simulink model "CR"  (R2022a)
settings: Solver=FixedStepDiscrete  StartTime=0.0  StopTime=1  FixedStep=0.04  RelTol=1e-3
PreLoadFcn:
  | listing = dir;
  | if (contains([listing .name], 'AGR')) && (contains([listing .name], 'MAP'))
  |     addpath('./AGR', './MAP');
  |     addpath( genpath('./MAP') );
  | elseif (contains([listing .name], 'CR.slx'))
  |     addpath('../AGR', '../MAP');
  |     addpath( genpath('../MAP') );
  | else
  | 
  | end
  | 
  | load('BusStructureCR.mat');
InitFcn:
  | listing = dir;
  | if (contains([listing .name], 'AGR')) && (contains([listing .name], 'MAP'))
  |     addpath('./AGR', './MAP');
  |     addpath( genpath('./MAP') );
  | elseif (contains([listing .name], 'CR.slx'))
  |     addpath('../AGR', '../MAP');
  |     addpath( genpath('../MAP') );
  | else
  | 
  | end
  | 
  | load('BusStructureCR.mat');
StartFcn:
  | listing = dir;
  | if (contains([listing .name], 'AGR')) && (contains([listing .name], 'MAP'))
  |     addpath('./AGR', './MAP');
  |     addpath( genpath('./MAP') );
  | elseif (contains([listing .name], 'CR.slx'))
  |     addpath('../AGR', '../MAP');
  |     addpath( genpath('../MAP') );
  | else
  | 
  | end
  | 
  | load('BusStructureCR.mat');
undefined symbols (not defined in the file or in its folder): CRDataTag, CRDataTagWrap, CRElevationValid, CRSelected, CRSelectedWraparound, CRTargetElevation, CRTargetLatitude, CRTargetLongitude, CRTargetLOSAvailable, CRTargetLOSAvailableValid, CRValid, deltaECEF, isFeasible, llh, losECEF, nSearch, targetECEF, testLLH
libraries: aerolibconvert2 x1
settings Model: Creator=ASCL  LastModifiedBy=ASCL
settings DataIOCC: SaveOutput=off  SignalLogging=off  DSMLogging=off  SaveTime=off  ReturnWorkspaceOutputs=off
settings OptimizationCC: BlockReduction=off  DefaultParameterBehavior=Inlined  UseDivisionForNetSlopeComputation=on  GainParamInheritBuiltInType=on  UseFloatMulNetSlope=on  ExpressionFolding=off  PassReuseOutputArgsAs=Individual arguments  ZeroExternalMemoryAtStartup=off  ZeroInternalMemoryAtStartup=off  NoFixptDivByZeroProtection=on  EfficientFloat2IntCast=on  LifeSpan=inf  OptimizeBlockOrder=speed  DifferentSizesBufferReuse=on  EfficientTunableParamExpr=on
settings DebuggingCC: SignalInfNanChecking=warning  ReadBeforeWriteMsg=EnableAllAsWarning  WriteAfterWriteMsg=EnableAllAsError  WriteAfterReadMsg=EnableAllAsError  IntegerOverflowMsg=error  ParameterTunabilityLossMsg=error  UniqueDataStoreMsg=error  AssertControl=DisableAll  NonBusSignalsTreatedAsBus=error  SFInvalidInputDataAccessInChartInitDiag=error  SFTransitionOutsideNaturalParentDiag=error  SFUnreachableExecutionPathDiag=error  SFUndirectedBroadcastEventsDiag=error  IntegerSaturationMsg=error
settings HardwareCC: ProdBitPerPointer=32  ProdBitPerSizeT=32  ProdBitPerPtrDiffT=32  ProdLargestAtomicInteger=Long  ProdLargestAtomicFloat=Double  ProdEndianess=BigEndian  ProdWordSize=32  ProdLongLongMode=on  ProdHWDeviceType=Freescale->MPC83xx
settings ModelReferenceCC: ModelReferenceNumInstancesAllowed=Single
settings SFSimCC: SimCustomHeaderCode="#include \"MAP.h\""  SimUserSources=MAP.c  SimUserLibraries=WS2_32.LIB  CompileTimeRecursionLimit=0  EnableRuntimeRecursion=off  MATLABDynamicMemAlloc=off
settings RTWCC: SystemTargetFile=ert.tlc  TemplateMakefile=ert_default_tmf  GenerateReport=on  RTWUseSimCustomCode=on  CustomHeaderCode="#include \"MAP.h\""  CustomSource=MAP.c  CustomLibrary=WS2_32.LIB  BuildConfiguration=Faster Runs  IncludeHyperlinkInReport=on  LaunchReport=on  GenerateTraceInfo=on  GenerateTraceReport=on  GenerateTraceReportSl=on  GenerateTraceReportSf=on  GenerateTraceReportEml=on  GenerateCodeMetricsReport=on
settings CodeAppCC: ForceParamTrailComments=on  IgnoreCustomStorageClasses=off  OperatorAnnotations=on  SimulinkDataObjDesc=on  SFDataObjDesc=on  MATLABFcnDesc=on  InsertBlockDesc=on  StateflowObjectComments=on  MATLABSourceComments=on  EnableCustomComments=on  InlinedPrmAccess=Macros  ReqsInCode=on
settings ERTTargetCC: TargetLangStandard=C99 (ISO)  UtilityFuncGeneration=Shared location  GenerateSampleERTMain=on  IncludeMdlTerminateFcn=off  CombineSignalStateStructs=on  SuppressErrorStatus=on  SupportAbsoluteTime=off  SupportNonFinite=off  SupportComplex=off  SupportVariableSizeSignals=on  ParenthesesLevel=Standards  CastingMode=Standards  GenerateSharedConstants=off  InlinedParameterPlacement=NonHierarchical  ERTCustomFileTemplate=example_file_process.tlc  RateTransitionBlockCode=Function  PreserveIfCondition=on  ConvertIfToSwitch=off  EnableSignedLeftShifts=off  EnableSignedRightShifts=off

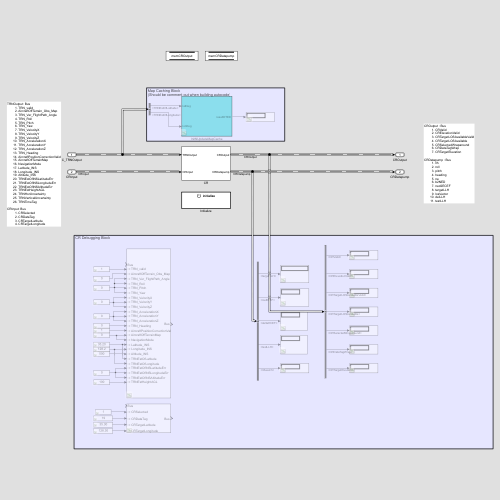
[thumbnail: Simulink's stored preview of the top-level diagram]
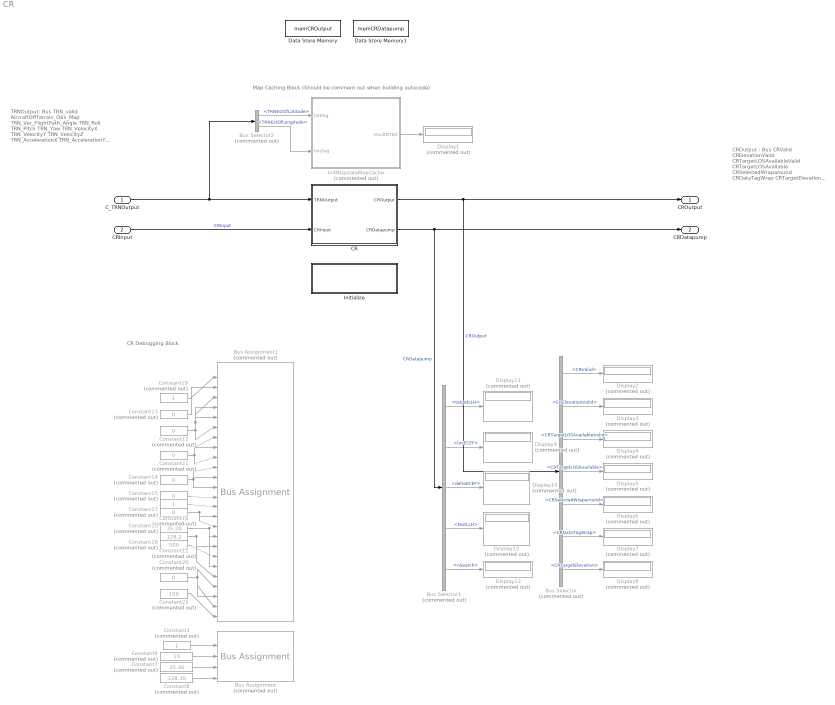
== system CR ==
  note: Map Caching Block
      | (Should be comment out when building autocode)
  note: TRNOutput: Bus
      | TRN_valid
      | AircraftOffTerrain_Obs_Map
      | TRN_Ver_FlightPath_Angle
      | TRN_Roll
      | TRN_Pitch
      | TRN_Yaw
      | TRN_VelocityX
      | TRN_VelocityY
      | TRN_VelocityZ
      | TRN_AccelerationX
      | TRN_AccelerationY
      | TRN_AccelerationZ
      | TRN_Heading
      | AircraftPositionCorrectionValid
      | AircraftOffTerrainMap
      | NavigationMode
      | Latitude_INS
      | Longitude_INS
      | Altitude_INS
      | TRNEstOfINSLatitudeErr
      | TRNEstOfINSLongitudeErr
      | TRNEstOfINSAltitudeErr
      | TRNEstHeightAGL
      | TRNHorUncertainty
      | TRNVerticalUncertainty
      | TRNTimeTag
      |
      | CRInput: Bus
      | CRSelected
      | CRDataTag
      | CRTargetLatitude
      | CRTargetLongitude
  note: CROutput : Bus
      | CRValid
      | CRElevationValid
      | CRTargetLOSAvailableValid
      | CRTargetLOSAvailable
      | CRSelectedWraparound
      | CRDataTagWrap
      | CRTargetElevation
      |
      | CRDatapump : Bus
      | llh
      | roll
      | pitch
      | heading
      | ne
      | b2NED
      | ned2ECEF
      | targetLLH
      | losVector
      | delLLH
      | testLLH
  note: CR Debugging Block
  C_TRNOutput : Inport  OutDataTypeStr=Bus: TRNOutput  Interpolate=off  BusOutputAsStruct=on
  CRInput : Inport  Port=2  OutDataTypeStr=Bus: CRInput  Interpolate=off  BusOutputAsStruct=on
  Bus Assignment : BusAssignment  Commented=on  AssignedSignals=CRSelected,CRDataTag,CRTargetLatitude,CRTargetLongitude
  Bus Assignment1 : BusAssignment  Commented=on  AssignedSignals=TRN_valid,AircraftOffTerrain_Obs_Map,TRN_Ver_FlightPath_Angle,TRN_Roll,TRN_Pitch,TRN_Yaw,TRN_VelocityX,TRN_VelocityY,TRN_VelocityZ,TRN_AccelerationX,TRN_AccelerationY,TRN_AccelerationZ,TRN_Heading,AircraftPositionCorrectionValid,AircraftOffTerrainMap,NavigationMode,Latitude_INS,Longitude_INS,Altitude_INS,TRNEstOfLatitude,TRNEstOfLongitude,TRNEstOfINSLatitudeErr,TRNEstOfINSLongitudeErr,TRNEstOfINSAltitudeErr,TRNEstHeightAGL
  Bus Selector : BusSelector  Commented=on  OutputSignals=CRValid,CRElevationValid,CRTargetLOSAvailableValid,CRTargetLOSAvailable,CRSelectedWraparound,CRDataTagWrap,CRTargetElevation
  Bus Selector1 : BusSelector  Commented=on  OutputSignals=targetLLH,losECEF,deltaECEF,testLLH,nSearch
  Bus Selector2 : BusSelector  Commented=on  OutputSignals=TRNEstOfLatitude,TRNEstOfLongitude
  CR : Subsystem
      mask init:
      | % latGPS = double(0);
      | % lonGPS = double(0);
      | % altGPS = double(0);
      | % velEGPS = double(0);
      | % velNGPS = double(0);
      | % velUGPS = double(0);
      | % notValidGPS = boolean(0);
      | % notAvaildINS = boolean(0);
      | % velUINS = double(0);
      | % velVINS = double(0);
      | % velWINS = double(0);
      | % rollINS = double(0);
      | % pitchINS = double(0);
      | % hgdINS = double(0);
      | % accXINS = double(0);
      | % accYINS = double(0);
      | % accZINS = double(0);
      | % activated = boolean(0);
      | % reactionT = uint16(0);
      | % pullUpG = uint16(0);
      | % rollRate = uint16(0);
      | % gOnsetRate = uint16(0);
      | % maxGamma = uint16(0);
      | % setWarnH = double(0);
      | % obsWarningTime = uint16(1);
      | % wiresWarningTime = uint16(1);
      | % latErrOfINS = double(0);
      | % lonErrOfINS = double(0);
      | % altErrorofINS = uint16(0);
      | % heightEstOfTRN = uint16(0);
      | % horUncertaintyOfTRN = double(0);
      | % verUncertaintyOfTRN = double(0);
  Constant10 : Constant  Commented=on  Value=35.20
  Constant11 : Constant  Commented=on  Value=128.2
  Constant{12,14..15,20..21} (5 alike) : Constant  Commented=on  Value=0
  Constant13 : Constant  Commented=on  Value=0  OutDataTypeStr=boolean
  Constant16 : Constant  Commented=on  OutDataTypeStr=boolean
  Constant17 : Constant  Commented=on  Value=0  OutDataTypeStr=boolean
  Constant18 : Constant  Commented=on  Value=500
  Constant19 : Constant  Commented=on  OutDataTypeStr=boolean
  Constant22 : Constant  Commented=on  Value=100  OutDataTypeStr=uint16
  Constant3 : Constant  Commented=on  OutDataTypeStr=boolean
  Constant7 : Constant  Commented=on  Value=35.30
  Constant8 : Constant  Commented=on  Value=128.30
  Constant9 : Constant  Commented=on  Value=19  OutDataTypeStr=uint16
  Data Store Memory : DataStoreMemory  DataStoreName=memCROutput  WriteAfterWriteMsg=warning  ShowAdditionalParam=off  OutDataTypeStr=Bus: CROutput
  Data Store Memory1 : DataStoreMemory  DataStoreName=memCRDatapump  WriteAfterWriteMsg=warning  ShowAdditionalParam=off  OutDataTypeStr=Bus: CRDatapump
  Display{1..13} (13 alike) : Display  Commented=on
  InitNUpdateMapCache : Subsystem  Commented=on  TreatAsAtomicUnit=on
  Initialize : Subsystem  TreatAsAtomicUnit=on
  CROutput : Outport  OutDataTypeStr=Bus: CROutput  VectorParamsAs1DForOutWhenUnconnected=off  BusOutputAsStruct=on
  CRDatapump : Outport  Port=2  OutDataTypeStr=Bus: CRDatapump  VectorParamsAs1DForOutWhenUnconnected=off  BusOutputAsStruct=on
  wires:
  CR/2(CRDatapump) -> Bus Selector1/1, CRDatapump/1  "CRDatapump"
  Constant16/1 -> Bus Assignment1/15
  Bus Selector1/4 -> Display12/1  "<testLLH>"
  Bus Selector/2 -> Display3/1  "<CRElevationValid>"
  CRInput/1 -> CR/2(CRInput)  "CRInput"
  Bus Selector1/2 -> Display9/1  "<losECEF>"
  Bus Selector1/5 -> Display13/1  "<nSearch>"
  Constant13/1 -> Bus Assignment1/3
  Bus Selector/6 -> Display7/1  "<CRDataTagWrap>"
  Constant17/1 -> Bus Assignment1/17, Bus Assignment1/16
  Constant9/1 -> Bus Assignment/3
  Bus Selector2/2 -> InitNUpdateMapCache/2(lonDeg)  "<TRNEstOfLongitude>"
  Bus Selector/4 -> Display5/1  "<CRTargetLOSAvailable>"
  Bus Selector/7 -> Display8/1  "<CRTargetElevation>"
  Constant12/1 -> Bus Assignment1/7, Bus Assignment1/4, Bus Assignment1/5, Bus Assignment1/6
  Bus Selector/5 -> Display6/1  "<CRSelectedWraparound>"
  Bus Selector/1 -> Display2/1  "<CRValid>"
  C_TRNOutput/1 -> Bus Selector2/1, CR/1(TRNOutput)
  Constant20/1 -> Bus Assignment1/23, Bus Assignment1/25, Bus Assignment1/24
  Constant14/1 -> Bus Assignment1/13, Bus Assignment1/11, Bus Assignment1/12
  Constant21/1 -> Bus Assignment1/10, Bus Assignment1/8, Bus Assignment1/9
  Bus Selector1/1 -> Display11/1  "<targetLLH>"
  Constant19/1 -> Bus Assignment1/2
  Bus Selector/3 -> Display4/1  "<CRTargetLOSAvailableValid>"
  Constant18/1 -> Bus Assignment1/20
  Constant10/1 -> Bus Assignment1/21, Bus Assignment1/18
  Constant8/1 -> Bus Assignment/5
  Bus Selector1/3 -> Display10/1  "<deltaECEF>"
  Constant7/1 -> Bus Assignment/4
  Constant3/1 -> Bus Assignment/2
  Constant22/1 -> Bus Assignment1/26
  Bus Selector2/1 -> InitNUpdateMapCache/1(latDeg)  "<TRNEstOfLatitude>"
  CR/1(CROutput) -> Bus Selector/1, CROutput/1  "CROutput"
  Constant11/1 -> Bus Assignment1/22, Bus Assignment1/19
  Constant15/1 -> Bus Assignment1/14
  InitNUpdateMapCache/1(resultDTED) -> Display1/1

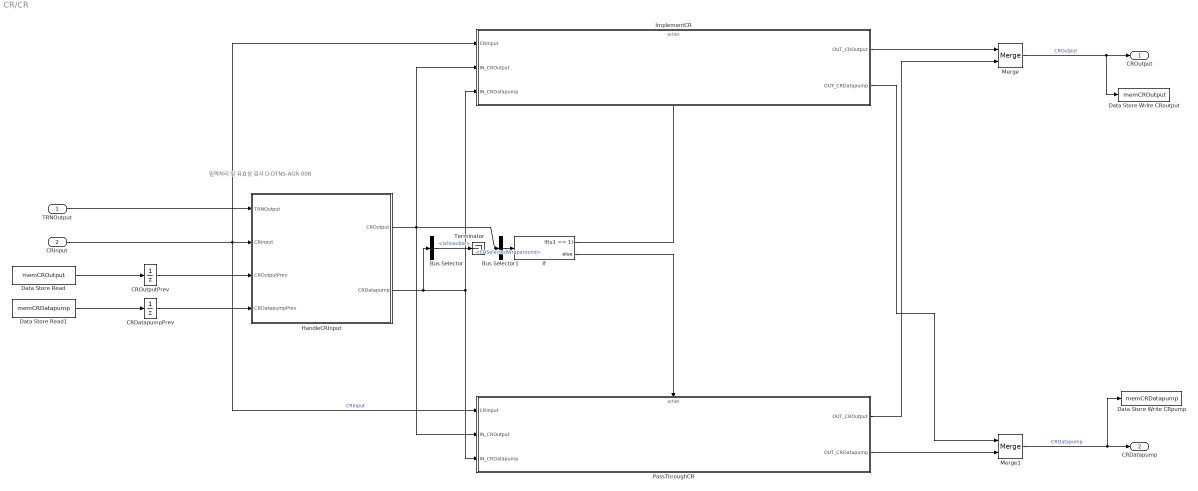
== system CR/CR ==
  note: 입력처리 및 유효성 검사 D-DTNS-AGR-008
  TRNOutput : Inport  OutDataTypeStr=Bus: TRNOutput
  CRInput : Inport  Port=2  OutDataTypeStr=Bus: CRInput
  Bus Selector : BusSelector  OutputSignals=isFeasible
  Bus Selector1 : BusSelector  OutputSignals=CRSelectedWraparound
  CRDatapumpPrev : UnitDelay  SampleTime=-1  HasFrameUpgradeWarning=on
  CROutputPrev : UnitDelay  SampleTime=-1  HasFrameUpgradeWarning=on
  Data Store Read : DataStoreRead  DataStoreName=memCROutput  IndexOptions=Index vector (dialog)  Indices=1  OutputSizes=1
  Data Store Read1 : DataStoreRead  DataStoreName=memCRDatapump  IndexOptions=Index vector (dialog)  Indices=1  OutputSizes=1
  Data Store Write CRoutput : DataStoreWrite  DataStoreName=memCROutput  IndexOptions=Index vector (dialog)  Indices=1  OutputSizes=1
  Data Store Write CRpump : DataStoreWrite  DataStoreName=memCRDatapump  IndexOptions=Index vector (dialog)  Indices=1  OutputSizes=1
  HandleCRInput : Subsystem  TreatAsAtomicUnit=on
      settings: RTWSystemCode=Nonreusable function  RTWFcnNameOpts=Use subsystem name
  If : If  IfExpression=u1 == 1
  ImplementCR : Subsystem  TreatAsAtomicUnit=on
      settings: RTWSystemCode=Nonreusable function  RTWFcnNameOpts=Use subsystem name
  Merge : Merge
  Merge1 : Merge
  PassThroughCR : Subsystem  TreatAsAtomicUnit=on
      settings: RTWSystemCode=Nonreusable function  RTWFcnNameOpts=Use subsystem name
  Terminator : Terminator
  CROutput : Outport  OutDataTypeStr=Bus: CROutput  VectorParamsAs1DForOutWhenUnconnected=off
  CRDatapump : Outport  Port=2  OutDataTypeStr=Bus: CRDatapump  VectorParamsAs1DForOutWhenUnconnected=off
  wires:
  CRInput/1 -> ImplementCR/1(CRInput), PassThroughCR/1(CRInput), HandleCRInput/2(CRInput)  "CRInput"
  Merge/1 -> CROutput/1, Data Store Write CRoutput/1  "CROutput"
  Merge1/1 -> Data Store Write CRpump/1, CRDatapump/1  "CRDatapump"
  Data Store Read/1 -> CROutputPrev/1
  Data Store Read1/1 -> CRDatapumpPrev/1
  ImplementCR/1(OUT_CROutput) -> Merge/1
  PassThroughCR/2(OUT_CRDatapump) -> Merge1/2
  ImplementCR/2(OUT_CRDatapump) -> Merge1/1
  PassThroughCR/1(OUT_CROutput) -> Merge/2
  HandleCRInput/1(CROutput) -> Bus Selector1/1, PassThroughCR/2(IN_CROutput), ImplementCR/2(IN_CROutput)
  HandleCRInput/2(CRDatapump) -> Bus Selector/1, PassThroughCR/3(IN_CRDatapump), ImplementCR/3(IN_CRDatapump)
  Bus Selector/1 -> Terminator/1  "<isFeasible>"
  If/1 -> ImplementCR/Action
  If/2 -> PassThroughCR/Action
  TRNOutput/1 -> HandleCRInput/1(TRNOutput)
  CROutputPrev/1 -> HandleCRInput/3(CROutputPrev)
  CRDatapumpPrev/1 -> HandleCRInput/4(CRDatapumpPrev)
  Bus Selector1/1 -> If/1  "<CRSelectedWraparound>"

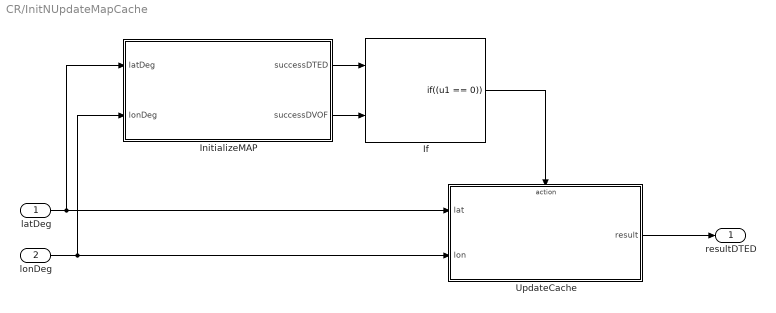
== system CR/InitNUpdateMapCache ==
  latDeg : Inport  OutDataTypeStr=double
  lonDeg : Inport  Port=2  OutDataTypeStr=double
  If : If  NumInputs=2  IfExpression=(u1 == 0)  ShowElse=off
  InitializeMAP : MATLAB Function  TreatAsAtomicUnit=on
  UpdateCache : Subsystem  TreatAsAtomicUnit=on
  resultDTED : Outport  VectorParamsAs1DForOutWhenUnconnected=off
  wires:
  lonDeg/1 -> InitializeMAP/2(lonDeg), UpdateCache/2(lon)
  UpdateCache/1(result) -> resultDTED/1
  InitializeMAP/1(successDTED) -> If/1
  latDeg/1 -> InitializeMAP/1(latDeg), UpdateCache/1(lat)
  InitializeMAP/2(successDVOF) -> If/2
  If/1 -> UpdateCache/Action

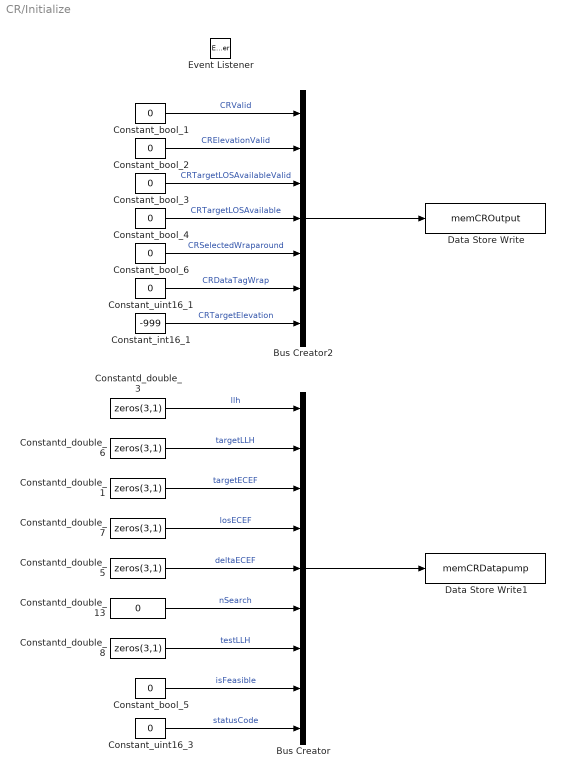
== system CR/Initialize ==
  Bus Creator : BusCreator  Inputs=9  OutDataTypeStr=Bus: CRDatapump  NonVirtualBus=on
  Bus Creator2 : BusCreator  Inputs=7  OutDataTypeStr=Bus: CROutput  NonVirtualBus=on
  Constant_bool_{1..6} (6 alike) : Constant  Value=0  OutDataTypeStr=boolean
  Constant_int16_1 : Constant  Value=-999  OutDataTypeStr=int16
  Constant_uint16_1 : Constant  Value=0  OutDataTypeStr=uint16
  Constant_uint16_3 : Constant  Value=0  OutDataTypeStr=uint16
  Constantd_double_{1,3,5..8} (6 alike) : Constant  Value=zeros(3,1)  OutDataTypeStr=double
  Constantd_double_13 : Constant  Value=0  OutDataTypeStr=double
  Data Store Write : DataStoreWrite  DataStoreName=memCROutput  IndexOptions=Index vector (dialog)  Indices=1  OutputSizes=1
  Data Store Write1 : DataStoreWrite  DataStoreName=memCRDatapump  IndexOptions=Index vector (dialog)  Indices=1  OutputSizes=1
  Event Listener : EventListener  DisableCoverage=on  EventName=reset
  wires:
  Bus Creator2/1 -> Data Store Write/1
  Constant_bool_4/1 -> Bus Creator2/4  "CRTargetLOSAvailable"
  Constant_bool_1/1 -> Bus Creator2/1  "CRValid"
  Constant_bool_2/1 -> Bus Creator2/2  "CRElevationValid"
  Constant_bool_3/1 -> Bus Creator2/3  "CRTargetLOSAvailableValid"
  Constantd_double_3/1 -> Bus Creator/1  "llh"
  Bus Creator/1 -> Data Store Write1/1
  Constant_int16_1/1 -> Bus Creator2/7  "CRTargetElevation"
  Constant_uint16_1/1 -> Bus Creator2/6  "CRDataTagWrap"
  Constant_bool_6/1 -> Bus Creator2/5  "CRSelectedWraparound"
  Constantd_double_6/1 -> Bus Creator/2  "targetLLH"
  Constantd_double_1/1 -> Bus Creator/3  "targetECEF"
  Constantd_double_7/1 -> Bus Creator/4  "losECEF"
  Constantd_double_5/1 -> Bus Creator/5  "deltaECEF"
  Constantd_double_13/1 -> Bus Creator/6  "nSearch"
  Constantd_double_8/1 -> Bus Creator/7  "testLLH"
  Constant_bool_5/1 -> Bus Creator/8  "isFeasible"
  Constant_uint16_3/1 -> Bus Creator/9  "statusCode"

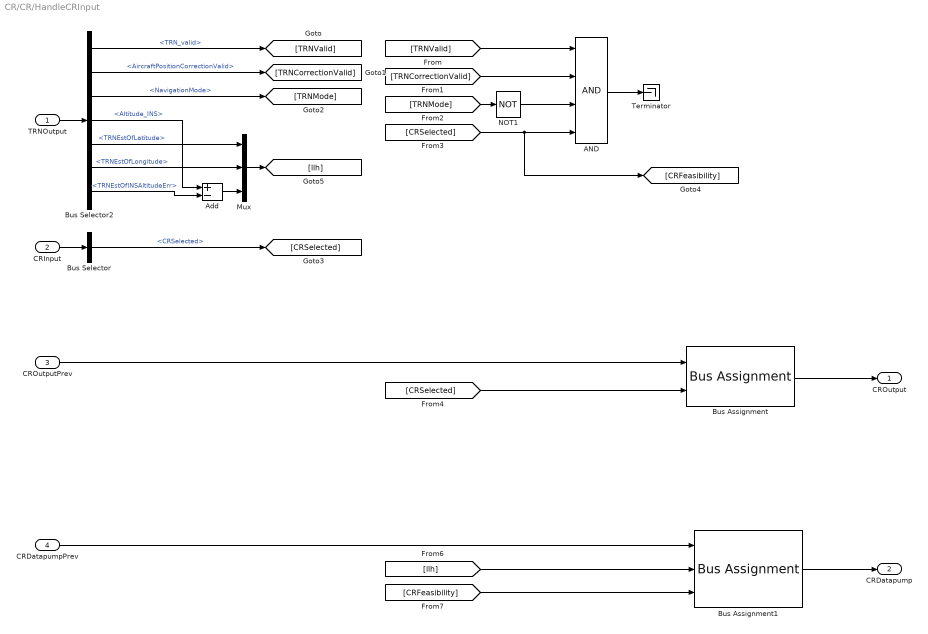
== system CR/CR/HandleCRInput ==
  TRNOutput : Inport  OutDataTypeStr=Bus: TRNOutput
  CRInput : Inport  Port=2  OutDataTypeStr=Bus: CRInput
  CROutputPrev : Inport  Port=3  OutDataTypeStr=Bus: CROutput
  CRDatapumpPrev : Inport  Port=4  OutDataTypeStr=Bus: CRDatapump
  AND : Logic  Inputs=4  AllPortsSameDT=off  OutDataTypeStr=boolean
  Add : Sum  Inputs=+-
  Bus Assignment : BusAssignment  AssignedSignals=CRSelectedWraparound
  Bus Assignment1 : BusAssignment  AssignedSignals=llh,isFeasible
  Bus Selector : BusSelector  OutputSignals=CRSelected
  Bus Selector2 : BusSelector  OutputSignals=TRN_valid,AircraftPositionCorrectionValid,NavigationMode,Altitude_INS,TRNEstOfLatitude,TRNEstOfLongitude,TRNEstOfINSAltitudeErr
  Mux : Mux  Inputs=3
  NOT1 : Logic  Operator=NOT  IconShape=distinctive  AllPortsSameDT=off  OutDataTypeStr=boolean
  Terminator : Terminator
  CROutput : Outport  OutDataTypeStr=Bus: CROutput  VectorParamsAs1DForOutWhenUnconnected=off
  CRDatapump : Outport  Port=2  OutDataTypeStr=Bus: CRDatapump  VectorParamsAs1DForOutWhenUnconnected=off
  wires:
  CRInput/1 -> Bus Selector/1
  CROutputPrev/1 -> Bus Assignment/1
  CRDatapumpPrev/1 -> Bus Assignment1/1
  Bus Selector/1 -> [CRSelected]  "<CRSelected>"
  TRNOutput/1 -> Bus Selector2/1
  Bus Selector2/2 -> [TRNCorrectionValid]  "<AircraftPositionCorrectionValid>"
  Bus Selector2/3 -> [TRNMode]  "<NavigationMode>"
  Bus Selector2/1 -> [TRNValid]  "<TRN_valid>"
  Bus Selector2/6 -> Mux/2  "<TRNEstOfLongitude>"
  Mux/1 -> [llh]
  Add/1 -> Mux/3
  Bus Selector2/5 -> Mux/1  "<TRNEstOfLatitude>"
  Bus Selector2/4 -> Add/1  "<Altitude_INS>"
  Bus Selector2/7 -> Add/2  "<TRNEstOfINSAltitudeErr>"
  [CRSelected] -> [CRFeasibility], AND/4
  NOT1/1 -> AND/3
  [TRNValid] -> AND/1
  [TRNCorrectionValid] -> AND/2
  [TRNMode] -> NOT1/1
  AND/1 -> Terminator/1
  Bus Assignment1/1 -> CRDatapump/1
  [llh] -> Bus Assignment1/2
  [CRFeasibility] -> Bus Assignment1/3
  Bus Assignment/1 -> CROutput/1
  [CRSelected] -> Bus Assignment/2

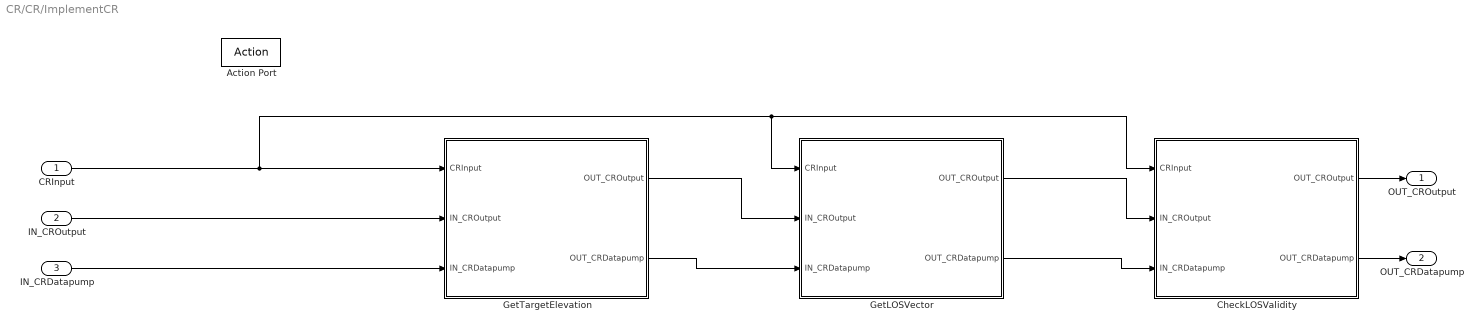
== system CR/CR/ImplementCR ==
  CRInput : Inport  OutDataTypeStr=Bus: CRInput
  IN_CROutput : Inport  Port=2  OutDataTypeStr=Bus: CROutput
  IN_CRDatapump : Inport  Port=3  OutDataTypeStr=Bus: CRDatapump
  Action Port : ActionPort  ActionPortLabel=if(u1 == 1)
  CheckLOSValidity : Subsystem  TreatAsAtomicUnit=on
      settings: RTWSystemCode=Nonreusable function  RTWFcnNameOpts=Use subsystem name
  GetLOSVector : Subsystem  TreatAsAtomicUnit=on
      settings: RTWSystemCode=Nonreusable function  RTWFcnNameOpts=Use subsystem name
  GetTargetElevation : Subsystem  TreatAsAtomicUnit=on
      settings: RTWSystemCode=Nonreusable function  RTWFcnNameOpts=Use subsystem name
  OUT_CROutput : Outport  OutDataTypeStr=Bus: CROutput  VectorParamsAs1DForOutWhenUnconnected=off
  OUT_CRDatapump : Outport  Port=2  OutDataTypeStr=Bus: CRDatapump  VectorParamsAs1DForOutWhenUnconnected=off
  wires:
  GetLOSVector/2(OUT_CRDatapump) -> CheckLOSValidity/3(IN_CRDatapump)
  IN_CRDatapump/1 -> GetTargetElevation/3(IN_CRDatapump)
  GetTargetElevation/2(OUT_CRDatapump) -> GetLOSVector/3(IN_CRDatapump)
  CRInput/1 -> CheckLOSValidity/1(CRInput), GetLOSVector/1(CRInput), GetTargetElevation/1(CRInput)
  IN_CROutput/1 -> GetTargetElevation/2(IN_CROutput)
  GetTargetElevation/1(OUT_CROutput) -> GetLOSVector/2(IN_CROutput)
  GetLOSVector/1(OUT_CROutput) -> CheckLOSValidity/2(IN_CROutput)
  CheckLOSValidity/1(OUT_CROutput) -> OUT_CROutput/1
  CheckLOSValidity/2(OUT_CRDatapump) -> OUT_CRDatapump/1

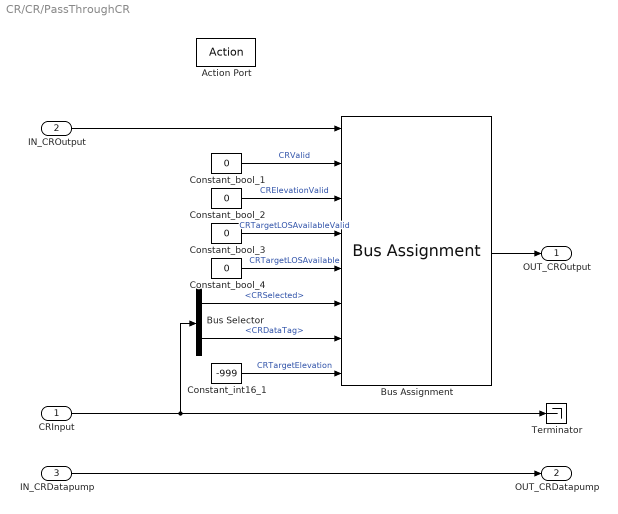
== system CR/CR/PassThroughCR ==
  CRInput : Inport  OutDataTypeStr=Bus: CRInput
  IN_CROutput : Inport  Port=2  OutDataTypeStr=Bus: CROutput
  IN_CRDatapump : Inport  Port=3  OutDataTypeStr=Bus: CRDatapump
  Action Port : ActionPort  ActionPortLabel=else
  Bus Assignment : BusAssignment  AssignedSignals=CRValid,CRElevationValid,CRTargetLOSAvailableValid,CRTargetLOSAvailable,CRSelectedWraparound,CRDataTagWrap,CRTargetElevation
  Bus Selector : BusSelector  OutputSignals=CRSelected,CRDataTag
  Constant_bool_{1..4} (4 alike) : Constant  Value=0  OutDataTypeStr=boolean
  Constant_int16_1 : Constant  Value=-999  OutDataTypeStr=int16
  Terminator : Terminator
  OUT_CROutput : Outport  OutDataTypeStr=Bus: CROutput  VectorParamsAs1DForOutWhenUnconnected=off
  OUT_CRDatapump : Outport  Port=2  OutDataTypeStr=Bus: CRDatapump  VectorParamsAs1DForOutWhenUnconnected=off
  wires:
  IN_CROutput/1 -> Bus Assignment/1
  IN_CRDatapump/1 -> OUT_CRDatapump/1
  CRInput/1 -> Bus Selector/1, Terminator/1
  Constant_bool_1/1 -> Bus Assignment/2  "CRValid"
  Bus Assignment/1 -> OUT_CROutput/1
  Bus Selector/2 -> Bus Assignment/7  "<CRDataTag>"
  Bus Selector/1 -> Bus Assignment/6  "<CRSelected>"
  Constant_bool_2/1 -> Bus Assignment/3  "CRElevationValid"
  Constant_bool_3/1 -> Bus Assignment/4  "CRTargetLOSAvailableValid"
  Constant_bool_4/1 -> Bus Assignment/5  "CRTargetLOSAvailable"
  Constant_int16_1/1 -> Bus Assignment/8  "CRTargetElevation"

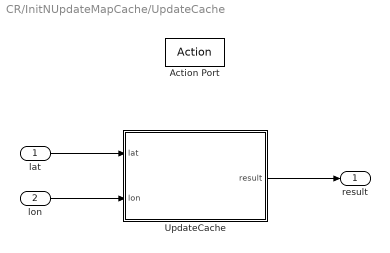
== system CR/InitNUpdateMapCache/UpdateCache ==
  lat : Inport
  lon : Inport  Port=2
  Action Port : ActionPort
  UpdateCache : MATLAB Function  TreatAsAtomicUnit=on
  result : Outport  VectorParamsAs1DForOutWhenUnconnected=off
  wires:
  UpdateCache/1(result) -> result/1
  lat/1 -> UpdateCache/1(lat)
  lon/1 -> UpdateCache/2(lon)

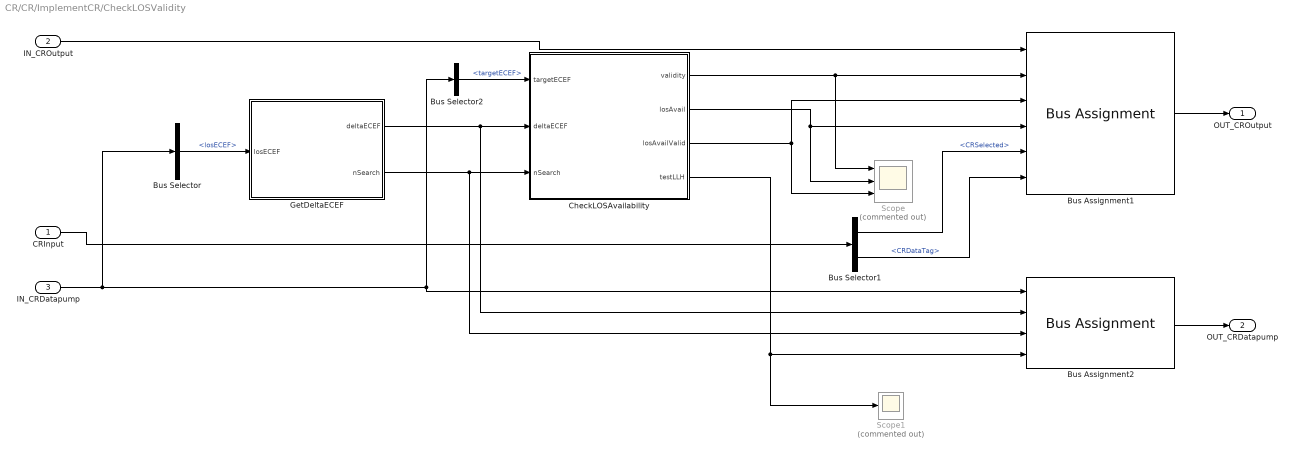
== system CR/CR/ImplementCR/CheckLOSValidity ==
  CRInput : Inport  OutDataTypeStr=Bus: CRInput
  IN_CROutput : Inport  Port=2  OutDataTypeStr=Bus: CROutput
  IN_CRDatapump : Inport  Port=3  OutDataTypeStr=Bus: CRDatapump
  Bus Assignment1 : BusAssignment  AssignedSignals=CRValid,CRTargetLOSAvailableValid,CRTargetLOSAvailable,CRSelectedWraparound,CRDataTagWrap
  Bus Assignment2 : BusAssignment  AssignedSignals=deltaECEF,nSearch,testLLH
  Bus Selector : BusSelector  OutputSignals=losECEF
  Bus Selector1 : BusSelector  OutputSignals=CRSelected,CRDataTag
  Bus Selector2 : BusSelector  OutputSignals=targetECEF
  CheckLOSAvailability : MATLAB Function  TreatAsAtomicUnit=on
      settings: RTWSystemCode=Nonreusable function  RTWFcnNameOpts=Use subsystem name  FunctionInterfaceSpec=Allow arguments (Match graphical interface)
  GetDeltaECEF : MATLAB Function  TreatAsAtomicUnit=on
  Scope : Scope  Commented=on  NumInputPorts=3
  Scope1 : Scope  Commented=on
  OUT_CROutput : Outport  OutDataTypeStr=Bus: CROutput  VectorParamsAs1DForOutWhenUnconnected=off
  OUT_CRDatapump : Outport  Port=2  OutDataTypeStr=Bus: CRDatapump  VectorParamsAs1DForOutWhenUnconnected=off
  wires:
  CRInput/1 -> Bus Selector1/1
  IN_CROutput/1 -> Bus Assignment1/1
  Bus Assignment1/1 -> OUT_CROutput/1
  IN_CRDatapump/1 -> Bus Selector2/1, Bus Assignment2/1, Bus Selector/1
  Bus Selector1/2 -> Bus Assignment1/6  "<CRDataTag>"
  CheckLOSAvailability/1(validity) -> Scope/1, Bus Assignment1/2
  CheckLOSAvailability/2(losAvail) -> Bus Assignment1/4, Scope/2
  CheckLOSAvailability/3(losAvailValid) -> Scope/3, Bus Assignment1/3
  Bus Assignment2/1 -> OUT_CRDatapump/1
  CheckLOSAvailability/4(testLLH) -> Bus Assignment2/4, Scope1/1
  Bus Selector/1 -> GetDeltaECEF/1(losECEF)  "<losECEF>"
  GetDeltaECEF/1(deltaECEF) -> CheckLOSAvailability/2(deltaECEF), Bus Assignment2/2
  GetDeltaECEF/2(nSearch) -> CheckLOSAvailability/3(nSearch), Bus Assignment2/3
  Bus Selector2/1 -> CheckLOSAvailability/1(targetECEF)  "<targetECEF>"
  Bus Selector1/1 -> Bus Assignment1/5  "<CRSelected>"

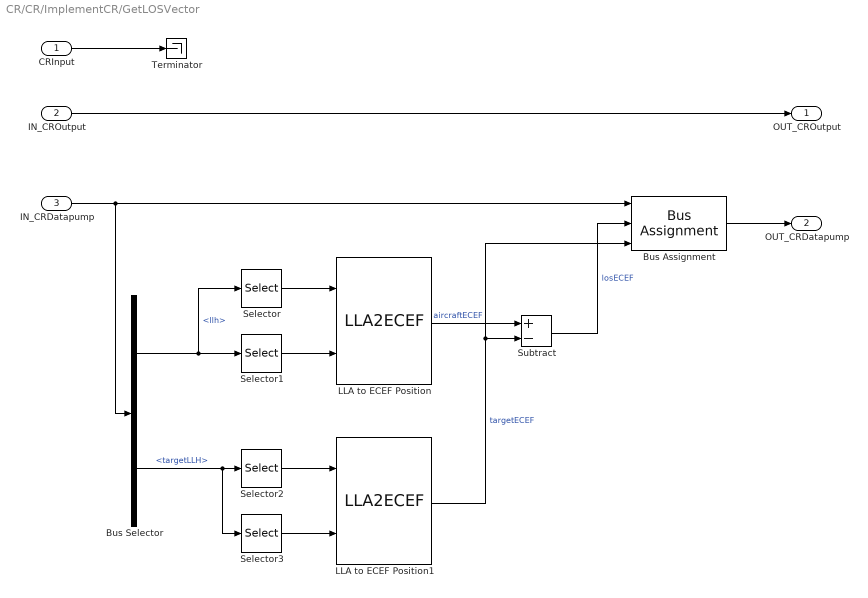
== system CR/CR/ImplementCR/GetLOSVector ==
  CRInput : Inport  OutDataTypeStr=Bus: CRInput
  IN_CROutput : Inport  Port=2  OutDataTypeStr=Bus: CROutput
  IN_CRDatapump : Inport  Port=3  OutDataTypeStr=Bus: CRDatapump
  Bus Assignment : BusAssignment  AssignedSignals=losECEF,targetECEF
  Bus Selector : BusSelector  OutputSignals=llh,targetLLH
  LLA to ECEF Position : LLA2ECEF
  LLA to ECEF Position1 : LLA2ECEF
  Selector : Selector  IndexMode=Zero-based  InputPortWidth=3  IndexOptions=Index vector (dialog)  Indices=[0 1]  OutputSizes=1
  Selector1 : Selector  IndexMode=Zero-based  InputPortWidth=3  IndexOptions=Index vector (dialog)  Indices=[2]  OutputSizes=1
  Selector2 : Selector  IndexMode=Zero-based  InputPortWidth=3  IndexOptions=Index vector (dialog)  Indices=[0 1]  OutputSizes=1
  Selector3 : Selector  IndexMode=Zero-based  InputPortWidth=3  IndexOptions=Index vector (dialog)  Indices=[2]  OutputSizes=1
  Subtract : Sum  Inputs=+-
  Terminator : Terminator
  OUT_CROutput : Outport  OutDataTypeStr=Bus: CROutput  VectorParamsAs1DForOutWhenUnconnected=off
  OUT_CRDatapump : Outport  Port=2  OutDataTypeStr=Bus: CRDatapump  VectorParamsAs1DForOutWhenUnconnected=off
  wires:
  IN_CRDatapump/1 -> Bus Selector/1, Bus Assignment/1
  CRInput/1 -> Terminator/1
  Bus Assignment/1 -> OUT_CRDatapump/1
  IN_CROutput/1 -> OUT_CROutput/1
  Bus Selector/1 -> Selector/1, Selector1/1  "<llh>"
  Bus Selector/2 -> Selector3/1, Selector2/1  "<targetLLH>"
  Subtract/1 -> Bus Assignment/2  "losECEF"
  Selector/1 -> LLA to ECEF Position/1
  Selector1/1 -> LLA to ECEF Position/2
  Selector2/1 -> LLA to ECEF Position1/1
  Selector3/1 -> LLA to ECEF Position1/2
  LLA to ECEF Position/1 -> Subtract/1  "aircraftECEF"
  LLA to ECEF Position1/1 -> Bus Assignment/3, Subtract/2  "targetECEF"

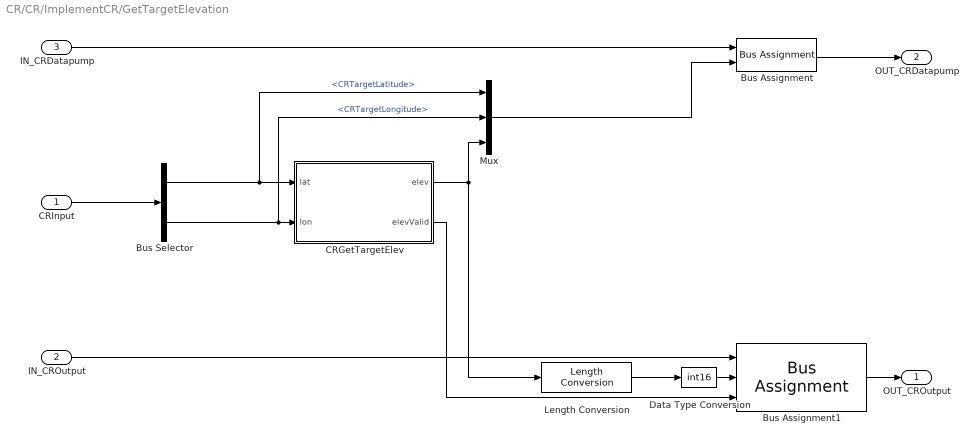
== system CR/CR/ImplementCR/GetTargetElevation ==
  CRInput : Inport  OutDataTypeStr=Bus: CRInput
  IN_CROutput : Inport  Port=2  OutDataTypeStr=Bus: CROutput
  IN_CRDatapump : Inport  Port=3  OutDataTypeStr=Bus: CRDatapump
  Bus Assignment : BusAssignment  AssignedSignals=targetLLH
  Bus Assignment1 : BusAssignment  AssignedSignals=CRTargetElevation,CRElevationValid
  Bus Selector : BusSelector  OutputSignals=CRTargetLatitude,CRTargetLongitude
  CRGetTargetElev : MATLAB Function  TreatAsAtomicUnit=on
  Data Type Conversion : DataTypeConversion  OutDataTypeStr=int16  RndMeth=Floor
  Length Conversion : aerolibconvert2/Length Conversion  IU=m  OU=ft
  Mux : Mux  Inputs=3
  OUT_CROutput : Outport  OutDataTypeStr=Bus: CROutput  VectorParamsAs1DForOutWhenUnconnected=off
  OUT_CRDatapump : Outport  Port=2  OutDataTypeStr=Bus: CRDatapump  VectorParamsAs1DForOutWhenUnconnected=off
  wires:
  IN_CRDatapump/1 -> Bus Assignment/1
  CRInput/1 -> Bus Selector/1
  Bus Selector/1 -> Mux/1, CRGetTargetElev/1(lat)  "<CRTargetLatitude>"
  Bus Selector/2 -> Mux/2, CRGetTargetElev/2(lon)  "<CRTargetLongitude>"
  CRGetTargetElev/1(elev) -> Length Conversion/1, Mux/3
  Mux/1 -> Bus Assignment/2
  Bus Assignment/1 -> OUT_CRDatapump/1
  IN_CROutput/1 -> Bus Assignment1/1
  Bus Assignment1/1 -> OUT_CROutput/1
  Data Type Conversion/1 -> Bus Assignment1/2
  CRGetTargetElev/2(elevValid) -> Bus Assignment1/3
  Length Conversion/1 -> Data Type Conversion/1

== matlab function CR/ImplementCR/GetTargetElevation/CRGetTargetElev ==
  data: lat input; elev output; lon input; elevValid output
function [elev, elevValid] = CRGetTargetElev(lat, lon)
%CRGetTargetElev

EPSILON = 0.001;

elev = 0.0;
elevValid = false;

elev = coder.ceval('MAPGetTerrainHeight', lat, lon);

% if (elev == -1.0)
if abs(elev - (-1.0)) < EPSILON
    elev = -999;
    elevValid = false;
else
    elevValid = true;
end

== matlab function CR/ImplementCR/CheckLOSValidity/GetDeltaECEF ==
  data: losECEF input; deltaECEF output; nSearch output
function [deltaECEF, nSearch] = GetDeltaECEF(losECEF)
%GetDeltaECEF
% 
% == Inputs =========
% losECEF           - LOS vector in {ECEF} [m]
% 
% == Outputs ========
% deltaECEF         - Incremental of LOS search vector in {ECEF} [m]
% nSearch           - number of intersection search required
% 

% Define
MIN_DIST = 30.0;

% Initialize
deltaECEF = zeros(3, 1);
nSearch = 2;

% Calculate the distance between A/C and target using los_ECEF vector
tarDistance = norm(losECEF);

% Calculate number of intersection search required
if (tarDistance < MIN_DIST)
    nSearch = 2;
else
    nSearch = ceil(tarDistance/MIN_DIST) + 1;
end

% Calculate the incremental of LOS search vector
deltaECEF = losECEF / (nSearch-1);

end

== matlab function CR/ImplementCR/CheckLOSValidity/CheckLOSAvailability ==
  data: targetECEF input; validity output; losAvail output; losAvailValid output; deltaECEF input; nSearch input; testLLH output
function [validity, losAvail, losAvailValid, testLLH] = CheckLOSAvailability(targetECEF, deltaECEF, nSearch)
%CheckLOSAvailability

% Initialization
validity        = true;
losAvail        = false;
losAvailValid   = false;
testLLH         = zeros(3, 1);
testElev        = 0.0;

EPSILON = 0.001;

for ii=1:(nSearch-1)

    % 1. Propagate search vector
    testECEF = targetECEF + (ii * deltaECEF); 
    
    % 2. Convert test ECEF coordinate to LLH
    testLLH = ConvertECEF2LLH(testECEF);

    % 3. Get & Test Terrain Elevation
    testElev = coder.ceval('MAPGetTerrainHeight', testLLH(1), testLLH(2));
    
%     if ( testElev == -1.0 )
    if abs(testElev-(-1.0)) < EPSILON
        losAvail = false;
        losAvailValid = false;
        return
    elseif (testElev > (testLLH(3)-1))
        losAvail = false;
        losAvailValid = true;
%         fprintf("LOS NOT AVAILABLE. Index: %f, testElev: %f, testLLH(3): %f \r\n", ii, testElev, testLLH(3));
        return
    else
        
    end

end

validity = true;
losAvail = true;
losAvailValid = true;

end

function llh  = ConvertECEF2LLH(xyzECEF)
%ConvertECEF2LLH
% Compute the {LLH} coordinates given {ECEF} coordinates
%
% == Inputs =========
% ecef              -  {ECEF} coordinates [m, m, m]
%
% == Outputs ========
% llh               - Corresponding Latitude, Longitude, Height [deg,deg,m]
%

% Initialize
llh = zeros(3,1);
lat     = 0.0;
lon     = 0.0;
h       = 0.0;

% WGS84 Parameters
r_e     = 6378137.0;            % major
f       = 1/298.257223563;      % (first) flattening
r_b     = r_e * (1-f);          % minor
e       = 0.08181919;           % Earth eccentricity
e2      = e*e;                  % Square of Earth eccentricity

% Rearrange
x       = xyzECEF(1);
y       = xyzECEF(2);
z       = xyzECEF(3);

% Longitude
lon = atan2d(y, x);

% Iteration for Latitude and Height [Bowring's method]

% Iteration parameters
eps     = 1;
tol     = 1e-12;

% side of triagle (hypotenuse: N+h, other side: z+N*e2*sind(lat) )
s       = sqrt(x^2 + y^2);

% Initial guesses
h   = 0.0;
N   = r_e;
lat = atand( z / (s * (1-e2*N/(N+h))) );

% Iteration terminates within 3~4 iterations.
count   = 0;

while (eps > tol) || (count > 10)
    lat0 = lat;

    % Recalculate
    h = s / cosd(lat) - N; 
    N   = r_e / sqrt(1-e2*(sind(lat))^2);
    lat = atand( z / (s * (1-e2*N/(N+h))) );

    % Update terminal condition parameters
    eps = abs(lat - lat0);
    count = count + 1;
end

llh = [lat; lon; h];

end

== matlab function CR/InitNUpdateMapCache/InitializeMAP ==
  data: successDTED output; successDVOF output; latDeg input; lonDeg input
function [successDTED, successDVOF] = InitializeMAP(latDeg, lonDeg)
%InitializeMAP

% Persistent variable
persistent firstRun
if isempty(firstRun)
    firstRun = true;
end

% Initialize output
flagDTED = int32(1);
flagDVOF = int32(1);
successDTED = int32(1);
successDVOF = int32(1);
hDEM = 0.0;

if firstRun
    % Path of DTED data
    pathDTED = 'C:\Users\ASCL\Documents\GitHub\DTNS\MAP\MAP_DB';

    % Length of DETD data path
    strLenDTED = int32(strlength(pathDTED));
    
    hDEM = coder.ceval('MAPGetTerrainHeight', latDeg, lonDeg);
    if IsNear(hDEM, -1.0)
        % Call [ InitialMap ] : 맵 폴더 위치 설정
        flagDTED = coder.ceval('InitialMap', pathDTED, strLenDTED );
        successDTED = flagDTED;
        if (~successDTED)
            firstRun = false;
        end
    else
        successDTED = int32(0);
        firstRun = false;       
    end
else
    successDTED = int32(0);
    successDVOF = int32(0);
end

== matlab function CR/InitNUpdateMapCache/UpdateCache/UpdateCache ==
  data: result output; lat input; lon input
function result = UpdateCache(lat, lon)
%UpdateCache

% Persistent variables
persistent latPrev lonPrev
if isempty(latPrev)
    latPrev = 0.0;
end
if isempty(lonPrev)
    lonPrev = 0.0;
end

% Initialize output
result = int32(1);

if ( abs(lat - latPrev) > 0.05 ) || ( abs(lon - lonPrev) > 0.05)
    result = coder.ceval('UpdateCache', lat, lon);
    latPrev = lat;
    lonPrev = lon;
else
    
end
